simulink model "Project2_Part2_sim"  (R2024b)
settings: Solver=VariableStepAuto  StartTime=0.0  StopTime=1000  RelTol=1e-3
undefined symbols (not defined in the file): carData, K_d, K_i, K_p
settings Model: NumberOfSteps=50  Creator=dxego  LastModifiedBy=mjsch
settings RTWCC: GPUComputeCapability=3.5

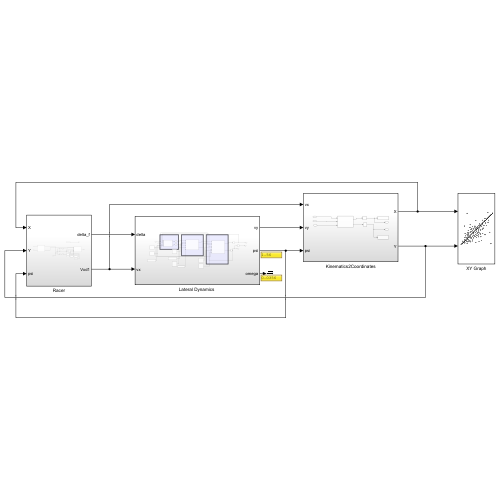
[thumbnail: Simulink's stored preview of the top-level diagram]
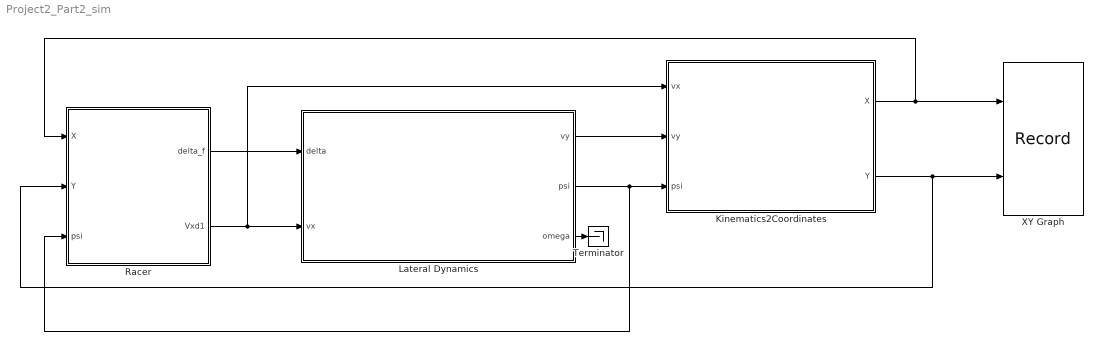
== system Project2_Part2_sim ==
  Kinematics2Coordinates : Subsystem
  "Lateral Dynamics " : Subsystem
  Racer : Subsystem
  Terminator : Terminator
  XY Graph : Record  FileSettingsInternal="{\"entries\":[{\"content\":{\"excelSettings\":{\"content\":{},\"type\":\"Streamout.ExcelSettings\"}},\"type\":\"Streamout.FileSettingStorage\",\"uuid\":\"\"}],\"packageUris\":[\"http:\\/\\/schema.mathworks.com\\/mf0\\/streamout_blocks\\/R2020a\"],\"version\":\"1.0\"}"  Layout=[1 1]  SignalsInternal="{\"entries\":[{\"content\":{\"signals\":[{\"content\":{\"blockPath\":[],\"dimensions\":[1],\"domain\":\"\",\"lineColor\":\"#4dbeee\",\"lineWidth\":2,\"port\":1,\"sid\":[\"\"],\"signalID\":1,\"signalName\":\"Kinematics2Coordinates:1\"},\"type\":\"RecordBlkView.Signal\",\"uuid\":\"\"},{\"content\":{\"blockPath\":[],\"dimensions\":[1],\"domain\":\"\",\"lineColor\":\"#edb120\",\"plots\":[ 1 ],\"port\":2,\"sid\":[\"\"],\"signalID\":2,\"signalName\":\"Kinematics2Coordinates:2\"},\"type\":\"RecordBlkView.Signal\",\"uuid\":\"\"}]},\"type\":\"RecordBlkView.InputSignals\",\"uuid\":\"\"}],\"packageUris\":[\"http:\\/\\/schema.mathworks.com\\/mf0\\/streamout_blocks\\/R2020a\"],\"version\":\"1.0\"}"  VisualizationBindings="{\"xyplotplugin\":{\"info\":[{\"series\":[{\"bindingParametersList\":[{\"parameter\":\"Y-Axis\",\"signalID\":2,\"signalName\":\"Kinematics2Coordinates:2\"}],\"seriesID\":0}],\"subplotID\":1}]}}"  CompatibilityTag=XY  st=-1
  wires:
  "Lateral Dynamics "/1(vy) -> Kinematics2Coordinates/2(vy)
  Kinematics2Coordinates/1(X) -> Racer/1(X), XY Graph/1
  Kinematics2Coordinates/2(Y) -> Racer/2(Y), XY Graph/2
  Racer/2(Vxd1) -> Kinematics2Coordinates/1(vx), "Lateral Dynamics "/2(vx)
  "Lateral Dynamics "/3(omega) -> Terminator/1
  Racer/1(delta_f) -> "Lateral Dynamics "/1(delta)
  "Lateral Dynamics "/2(psi) -> Racer/3(psi), Kinematics2Coordinates/3(psi)

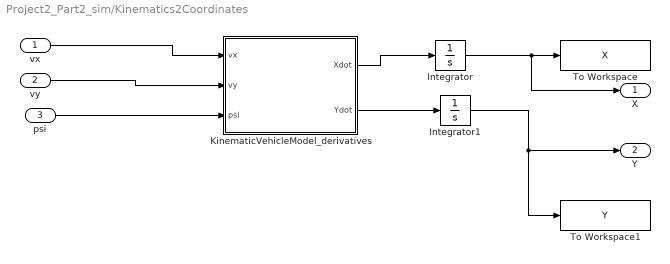
== system Project2_Part2_sim/Kinematics2Coordinates ==
  vx : Inport
  vy : Inport  Port=2
  psi : Inport  Port=3
  Integrator : Integrator  InitialCondition=carData.init.X0
  Integrator1 : Integrator  InitialCondition=carData.init.Y0
  KinematicVehicleModel_derivatives : MATLAB Function  TreatAsAtomicUnit=on
  To Workspace : ToWorkspace  VariableName=X  SaveFormat=Timeseries  SampleTime=-1
  To Workspace1 : ToWorkspace  VariableName=Y  SaveFormat=Timeseries  SampleTime=-1
  X : Outport
  Y : Outport  Port=2
  wires:
  Integrator/1 -> X/1, To Workspace/1
  Integrator1/1 -> To Workspace1/1, Y/1
  vx/1 -> KinematicVehicleModel_derivatives/1(vx)
  vy/1 -> KinematicVehicleModel_derivatives/2(vy)
  psi/1 -> KinematicVehicleModel_derivatives/3(psi)
  KinematicVehicleModel_derivatives/1(Xdot) -> Integrator/1
  KinematicVehicleModel_derivatives/2(Ydot) -> Integrator1/1

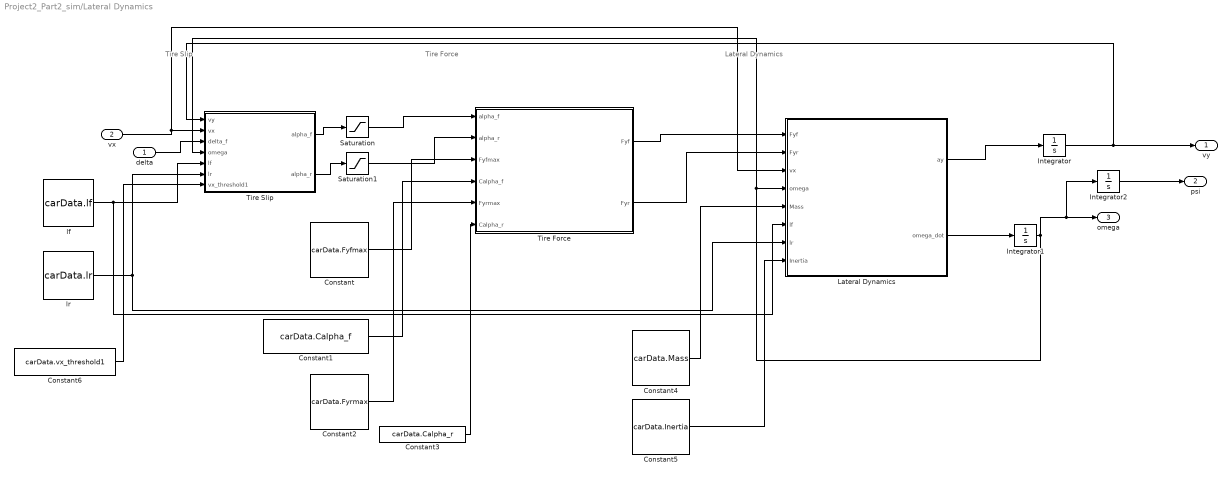
== system Project2_Part2_sim/Lateral Dynamics  ==
  note: Tire Slip
  note: Tire Force
  note: Lateral Dynamics
  delta : Inport
  vx : Inport  Port=2
  Constant : Constant  Value=carData.Fyfmax
  Constant1 : Constant  Value=carData.Calpha_f
  Constant2 : Constant  Value=carData.Fyrmax
  Constant3 : Constant  Value=carData.Calpha_r
  Constant4 : Constant  Value=carData.Mass
  Constant5 : Constant  Value=carData.Inertia
  Constant6 : Constant  Value=carData.vx_threshold1
  Integrator : Integrator  InitialCondition=carData.init.vy0
  Integrator1 : Integrator  InitialCondition=carData.init.omega0
  Integrator2 : Integrator  InitialCondition=carData.init.psi0  WrappedStateUpperValue=2*pi  WrappedStateLowerValue=0
  Lateral Dynamics : MATLAB Function  TreatAsAtomicUnit=on
  Saturation : Saturate  UpperLimit=carData.maxAlpha  LowerLimit=-carData.maxAlpha
  Saturation1 : Saturate  UpperLimit=carData.maxAlpha  LowerLimit=-carData.maxAlpha
  Tire Force : MATLAB Function  TreatAsAtomicUnit=on
  "Tire Slip " : MATLAB Function  TreatAsAtomicUnit=on
  lf : Constant  Value=carData.lf
  lr : Constant  Value=carData.lr
  vy : Outport
  psi : Outport  Port=2
  omega : Outport  Port=3
  wires:
  Lateral Dynamics/1(ay) -> Integrator/1
  Integrator/1 -> "Tire Slip "/1(vy), vy/1
  Lateral Dynamics/2(omega_dot) -> Integrator1/1
  Integrator1/1 -> Integrator2/1, omega/1, Lateral Dynamics/4(omega), "Tire Slip "/4(omega)
  "Tire Slip "/1(alpha_f) -> Saturation/1
  Saturation/1 -> Tire Force/1(alpha_f)
  Saturation1/1 -> Tire Force/2(alpha_r)
  vx/1 -> Lateral Dynamics/3(vx), "Tire Slip "/2(vx)
  delta/1 -> "Tire Slip "/3(delta_f)
  Integrator2/1 -> psi/1
  "Tire Slip "/2(alpha_r) -> Saturation1/1
  Tire Force/1(Fyf) -> Lateral Dynamics/1(Fyf)
  Tire Force/2(Fyr) -> Lateral Dynamics/2(Fyr)
  lf/1 -> Lateral Dynamics/6(lf), "Tire Slip "/5(lf)
  lr/1 -> Lateral Dynamics/7(lr), "Tire Slip "/6(lr)
  Constant/1 -> Tire Force/3(Fyfmax)
  Constant1/1 -> Tire Force/4(Calpha_f)
  Constant2/1 -> Tire Force/5(Fyrmax)
  Constant3/1 -> Tire Force/6(Calpha_r)
  Constant4/1 -> Lateral Dynamics/5(Mass)
  Constant5/1 -> Lateral Dynamics/8(Inertia)
  Constant6/1 -> "Tire Slip "/7(vx_threshold1)

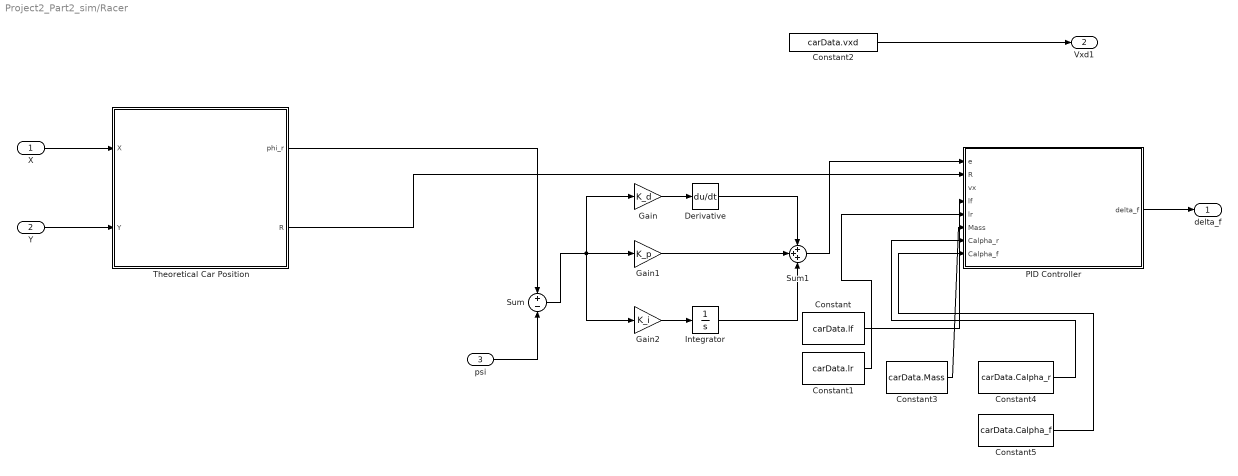
== system Project2_Part2_sim/Racer ==
  X : Inport
  Y : Inport  Port=2
  psi : Inport  Port=3
  Constant : Constant  Value=carData.lf
  Constant1 : Constant  Value=carData.lr
  Constant2 : Constant  Value=carData.vxd
  Constant3 : Constant  Value=carData.Mass
  Constant4 : Constant  Value=carData.Calpha_r
  Constant5 : Constant  Value=carData.Calpha_f
  Derivative : Derivative
  Gain : Gain  Gain=K_d
  Gain1 : Gain  Gain=K_p
  Gain2 : Gain  Gain=K_i
  Integrator : Integrator
  PID Controller : MATLAB Function  TreatAsAtomicUnit=on
  Sum : Sum  Inputs=+-
  Sum1 : Sum  Inputs=+++
  Theoretical Car Position : MATLAB Function  TreatAsAtomicUnit=on
  delta_f : Outport
  Vxd1 : Outport  Port=2
  wires:
  Constant2/1 -> Vxd1/1
  Y/1 -> Theoretical Car Position/2(Y)
  psi/1 -> Sum/2
  Gain/1 -> Derivative/1
  Gain2/1 -> Integrator/1
  Sum/1 -> Gain2/1, Gain/1, Gain1/1
  Derivative/1 -> Sum1/1
  Gain1/1 -> Sum1/2
  Integrator/1 -> Sum1/3
  Sum1/1 -> PID Controller/1(e)
  X/1 -> Theoretical Car Position/1(X)
  Constant/1 -> PID Controller/4(lf)
  Constant1/1 -> PID Controller/5(lr)
  Constant3/1 -> PID Controller/6(Mass)
  Constant4/1 -> PID Controller/7(Calpha_r)
  Constant5/1 -> PID Controller/8(Calpha_f)
  Theoretical Car Position/1(phi_r) -> Sum/1
  Theoretical Car Position/2(R) -> PID Controller/2(R)
  PID Controller/1(delta_f) -> delta_f/1

== matlab function Project2_Part2_sim/Lateral Dynamics /Tire Slip  ==
  data: vy input; alpha_f output; vx input; delta_f input; omega input; lf input; alpha_r output; lr input; vx_threshold1 input
function [alpha_f, alpha_r] = fcn(vy,  vx, delta_f, omega, lf, lr, vx_threshold1)


if abs(vx)> vx_threshold1
      alpha_f = delta_f - (vy + omega * lf) / vx;
      alpha_r = - (vy - omega * lr) / vx;
else
      alpha_f = 0;
      alpha_r = 0;
end



end

== matlab function Project2_Part2_sim/Racer/Theoretical Car Position ==
  data: X input; phi_r output; Y input; R output
function [phi_r, R] = car_position(X, Y)
    phi_r = 0;
    R = 0;
    
    if Y < 200
        if X >= 0 && X <= 900
            phi_r = 0; %first straight path from origin
            R = 0;
        elseif X > 900
            phi_r = 2*pi - acos((X - 900) / 200) - deg2rad(270); %first turn 
            R = 200;
        elseif X < 0
            phi_r = acos(-X / 200) + deg2rad(270); %turn 4
            R = 200;
        end
    else

        if X >= 0 && X <= 900
            phi_r = pi;
            R = 0;
        elseif X > 900
            phi_r = acos((X - 900) / 200) + deg2rad(90);
            R = 200;
        elseif X < 0
            phi_r = 2*pi - acos(-X / 200) - deg2rad(90);
            R = 200;

        end
    end
end

== matlab function Project2_Part2_sim/Kinematics2Coordinates/KinematicVehicleModel_derivatives ==
  data: vx input; Xdot output; vy input; psi input; Ydot output
function [Xdot, Ydot] = fcn(vx, vy, psi)
    temp = TF(psi) * [vx;vy]; 
    Xdot = temp(1);
    Ydot = temp(2);
  
end

function y = TF(psi)
    y = [cos(psi), -sin(psi); sin(psi), cos(psi)];
end

== matlab function Project2_Part2_sim/Lateral Dynamics /Tire Force ==
  data: alpha_f input; Fyf output; alpha_r input; Fyfmax input; Fyr output; Calpha_f input; Fyrmax input; Calpha_r input
function [Fyf, Fyr] = fcn(alpha_f, alpha_r, Fyfmax, Calpha_f, Fyrmax, Calpha_r)

Fyf = min(Fyfmax,Calpha_f * alpha_f);
Fyr = min(Fyrmax, Calpha_r * alpha_r);

end

== matlab function Project2_Part2_sim/Lateral Dynamics /Lateral Dynamics ==
  data: Fyf input; ay output; Fyr input; vx input; omega input; Mass input; omega_dot output; lf input; lr input; Inertia input
function [ay, omega_dot] = fcn(Fyf, Fyr, vx, omega, Mass, lf, lr, Inertia)

Fy = Fyf + Fyr;
ay = Fy / Mass - omega * vx;
        
M  = Fyf * lf - Fyr *lr;        
omega_dot = M / Inertia;        

end

== matlab function Project2_Part2_sim/Racer/PID Controller ==
  data: e input; delta_f output; R input; vx input; lf input; lr input; Mass input; Calpha_r input; Calpha_f input
function delta_f = fcn(e, R, vx, lf, lr, Mass, Calpha_r, Calpha_f)
L = lr + lf;
if R ~= 0
    delta_f = e + (L/R)+((Mass/(L*R))*((lr/Calpha_r)-(lf/Calpha_f))*(vx^2));
else
    delta_f = e;

end
